simulink model "chap4_10sim"  (Simulink 5.0)
settings: Solver=ode45  StartTime=0.0  StopTime=5  FixedStep=0.001  RelTol=1e-3
settings Model: LastModifiedBy=Administrator  ExtModeTrigMode=oneshot  ExtModeArmWhenConnect=off  LimitDataPoints=off  BooleanDataType=off

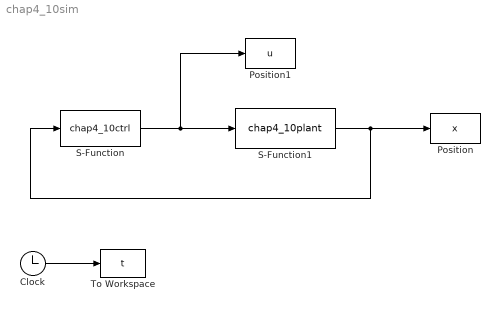
== system chap4_10sim ==
  Clock : Clock
      settings: Decimation=10
  Position : ToWorkspace  VariableName=x  SampleTime=-1  SaveFormat=Array
  Position1 : ToWorkspace  VariableName=u  SampleTime=-1  SaveFormat=Array
  S-Function : S-Function  FunctionName=chap4_10ctrl
  S-Function1 : S-Function  FunctionName=chap4_10plant
  To Workspace : ToWorkspace  VariableName=t  SampleTime=-1  SaveFormat=Array
  wires:
  S-Function/1 -> S-Function1/1, Position1/1
  S-Function1/1 -> S-Function/1, Position/1
  Clock/1 -> To Workspace/1
